simulink model "MyPTControlOSM_RTW"  (Simulink 8.7)
settings: Solver=ode1  SolverMode=SingleTasking  StartTime=0.0  StopTime=inf  FixedStep=0.0002  RelTol=1e-3
PreLoadFcn:
  | vehicle = 'Car'; if ~length(which('cmcmd')), cmenv; end
  | MyPTControlOSM_RTW_bus
InitFcn:
  | vehicle = 'Car'; if ~length(which('cmcmd')), cmenv; end
  | MyPTControlOSM_RTW_bus
undefined symbols (not defined in the file or in its folder): OperationState, OSMFunc, rv, State
libraries: simulink x14
(part 1 of 2)
Description:
  | CarMaker Plug-in Model Target
settings Model: Creator=ml  LastModifiedBy=IPG
settings DataIOCC: SignalLoggingSaveFormat=ModelDataLogs
settings OptimizationCC: ExpressionDepthLimit=2147483647
settings DebuggingCC: FcnCallInpInsideContextMsg=UseLocalSettings  StateNameClashWarn=warning
settings HardwareCC: TargetHWDeviceType=32-bit Generic  ProdEqTarget=off
settings RTWCC: SystemTargetFile=CarMaker.tlc  TemplateMakefile=CarMaker_unix-win64.tmf  Description=CarMaker Plug-in Model Target
settings CodeAppCC: MaxIdLength=63
settings STFCustomTargetCC: ModelReferenceCompliant=off  GeneratePreprocessorConditionals=Disable all  MultiInstanceERTCode=on  CodeInterfacePackaging=Reusable function  CPPClassGenCompliant=on  GRTInterface=off  GenerateAllocFcn=on  SystemTargetFile=CarMaker.tlc
settings GRTTargetCC: ModelReferenceCompliant=off  ParMdlRefBuildCompliant=off  CompOptLevelCompliant=off  ConcurrentExecutionCompliant=off  CombineOutputUpdateFcns=off  MatFileLogging=off  MultiInstanceERTCode=on  CodeInterfacePackaging=Reusable function  GenerateAllocFcn=on  UseToolchainInfoCompliant=off  ExtModeMexFile=noextcomm
settings CustomProperty: DataType=string  Value=..
settings EnumStrPairs: String=Car

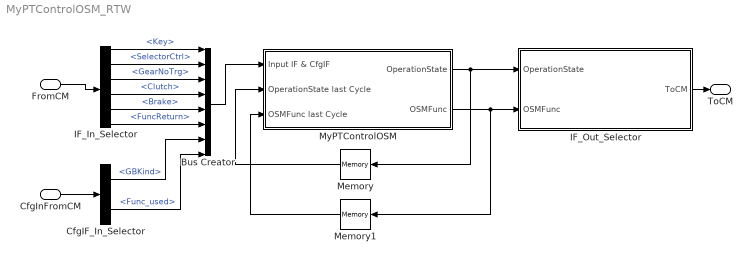
== system MyPTControlOSM_RTW ==
  FromCM : Inport  OutDataTypeStr=Bus: cmPTControlOSMIn
  CfgInFromCM : Inport  Port=2  OutDataTypeStr=Bus: cmPTControlOSMCfgIn
  Bus Creator : BusCreator  Inputs=8
  CfgIF_In_Selector : BusSelector  OutputSignals=GBKind,Func_used
  IF_In_Selector : BusSelector  OutputSignals=Key,SelectorCtrl,GearNoTrg,Clutch,Brake,FuncReturn
  IF_Out_Selector : Subsystem  mask(Signal Selection){}
      mask help: Signal Selection Block
      settings: OpenFcn=cmSignalSelect('SignalSelection_CB',gcb)
  Memory : Memory
  Memory1 : Memory
  MyPTControlOSM : Subsystem
  ToCM : Outport  OutDataTypeStr=Bus: cmPTControlOSMOut
  wires:
  FromCM/1 -> IF_In_Selector/1
  IF_Out_Selector/1(ToCM) -> ToCM/1
  CfgInFromCM/1 -> CfgIF_In_Selector/1
  MyPTControlOSM/1(OperationState) -> Memory/1, IF_Out_Selector/1(OperationState)
  Memory/1 -> MyPTControlOSM/2(OperationState last Cycle)
  IF_In_Selector/1 -> Bus Creator/1  "<Key>"
  IF_In_Selector/2 -> Bus Creator/2  "<SelectorCtrl>"
  IF_In_Selector/3 -> Bus Creator/3  "<GearNoTrg>"
  IF_In_Selector/4 -> Bus Creator/4  "<Clutch>"
  IF_In_Selector/5 -> Bus Creator/5  "<Brake>"
  IF_In_Selector/6 -> Bus Creator/6  "<FuncReturn>"
  CfgIF_In_Selector/1 -> Bus Creator/7  "<GBKind>"
  CfgIF_In_Selector/2 -> Bus Creator/8  "<Func_used>"
  Bus Creator/1 -> MyPTControlOSM/1(Input IF & CfgIF)
  Memory1/1 -> MyPTControlOSM/3(OSMFunc last Cycle)
  MyPTControlOSM/2(OSMFunc) -> Memory1/1, IF_Out_Selector/2(OSMFunc)

== system MyPTControlOSM_RTW/IF_Out_Selector ==
  OperationState : Inport
  OSMFunc : Inport  Port=2
  OperationError : Constant  Value=0
  RateTransition : RateTransition  OutPortSampleTime=str2num(get_param(bdroot,'FixedStep'))
  cmPTControlOSMOut : BusCreator  Inputs=3
  ToCM : Outport
  wires:
  RateTransition/1 -> ToCM/1
  cmPTControlOSMOut/1 -> RateTransition/1
  OperationError/1 -> cmPTControlOSMOut/2  "OperationError"
  OperationState/1 -> cmPTControlOSMOut/1  "OperationState"
  OSMFunc/1 -> cmPTControlOSMOut/3  "OSMFunc"

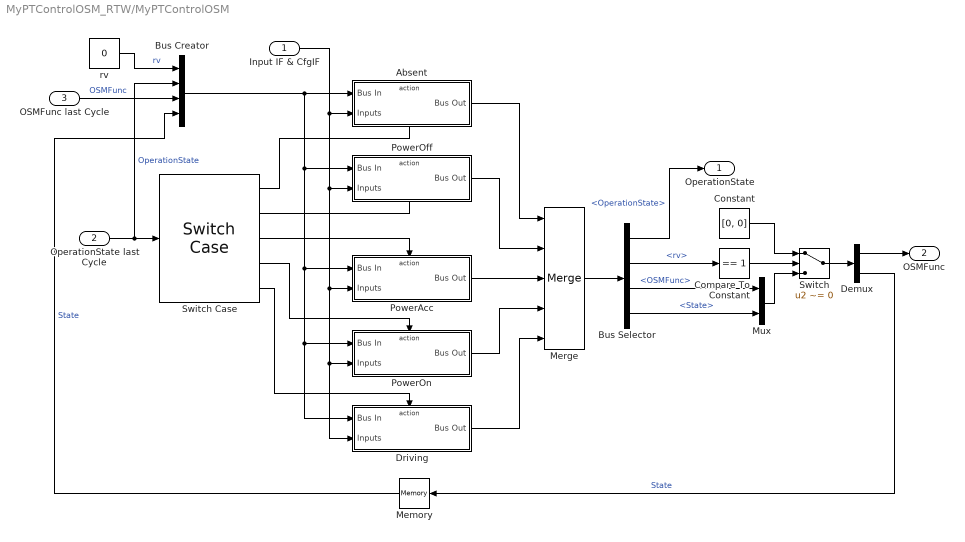
== system MyPTControlOSM_RTW/MyPTControlOSM ==
  Input IF & CfgIF : Inport
  OperationState last Cycle : Inport  Port=2
  OSMFunc last Cycle : Inport  Port=3
  Absent : Subsystem  TreatAsAtomicUnit=on
  Bus Creator : BusCreator  Inputs=4
  Bus Selector : BusSelector  OutputSignals=OperationState,rv,OSMFunc,State
  Compare To Constant : simulink/Logic and Bit Operations/Compare To Constant  SystemSampleTime=-1  relop===  const=1  LogicOutDataTypeMode=uint8  ZeroCross=off
  Constant : Constant  Value=[0, 0]
  Demux : Demux  Outputs=2
  Driving : Subsystem  TreatAsAtomicUnit=on
  Memory : Memory
  Merge : Merge  Inputs=5
  Mux : Mux  Inputs=2
  PowerAcc : Subsystem  TreatAsAtomicUnit=on
  PowerOff : Subsystem  TreatAsAtomicUnit=on
  PowerOn : Subsystem  TreatAsAtomicUnit=on
  Switch : Switch  Criteria=u2 ~= 0
  Switch Case : SwitchCase  CaseConditions={0,1,2,3}
  rv : Constant  Value=0
  OperationState : Outport
  OSMFunc : Outport  Port=2
  wires:
  OperationState last Cycle/1 -> Switch Case/1, Bus Creator/2  "OperationState"
  Switch Case/3 -> PowerAcc/Action
  Switch Case/2 -> PowerOff/Action
  Absent/1(Bus Out) -> Merge/1
  PowerOff/1(Bus Out) -> Merge/2
  PowerAcc/1(Bus Out) -> Merge/3
  rv/1 -> Bus Creator/1  "rv"
  Bus Creator/1 -> Absent/1(Bus In), PowerOff/1(Bus In), PowerAcc/1(Bus In), Driving/1(Bus In), PowerOn/1(Bus In)
  Merge/1 -> Bus Selector/1
  Input IF & CfgIF/1 -> PowerAcc/2(Inputs), Driving/2(Inputs), PowerOn/2(Inputs), PowerOff/2(Inputs), Absent/2(Inputs)
  Bus Selector/1 -> OperationState/1  "<OperationState>"
  Switch/1 -> Demux/1
  Demux/2 -> Memory/1  "State"
  Demux/1 -> OSMFunc/1
  Bus Selector/2 -> Compare To Constant/1  "<rv>"
  Bus Selector/3 -> Mux/1  "<OSMFunc>"
  Bus Selector/4 -> Mux/2  "<State>"
  OSMFunc last Cycle/1 -> Bus Creator/3  "OSMFunc"
  Memory/1 -> Bus Creator/4  "State"
  Driving/1(Bus Out) -> Merge/5
  PowerOn/1(Bus Out) -> Merge/4
  Compare To Constant/1 -> Switch/2
  Constant/1 -> Switch/1
  Mux/1 -> Switch/3
  Switch Case/4 -> PowerOn/Action
  Switch Case/5 -> Driving/Action
  Switch Case/1 -> Absent/Action

== system MyPTControlOSM_RTW/MyPTControlOSM/Absent ==
  Bus In : Inport
  Inputs : Inport  Port=2
  Absent : ActionPort  ActionType=case
  "Absent -> PowerOff?" : Subsystem  TreatAsAtomicUnit=on
  Absent Function exist? : Subsystem  TreatAsAtomicUnit=on
  Bus Selector : BusSelector  OutputSignals=State
  Merge : Merge  Inputs=6
  PowerOff function exist? : Subsystem  TreatAsAtomicUnit=on
  PowerOff reached : Subsystem  TreatAsAtomicUnit=on
  Signal Conversion : SignalConversion  ConversionOutput=Bus copy  OverrideOpt=off
  Switch Case : SwitchCase  CaseConditions={0,1,2,3,4}
  Wait for Absent is ready : Subsystem  TreatAsAtomicUnit=on
  Wait for PowerOff is ready : Subsystem  TreatAsAtomicUnit=on
  Bus Out : Outport
  wires:
  Signal Conversion/1 -> Bus Out/1
  Bus In/1 -> Bus Selector/1, Absent Function exist?/2(Bus In), Wait for Absent is ready/1(Bus In), "Absent -> PowerOff?"/1(Bus In), PowerOff reached/1(Bus In), Wait for PowerOff is ready/1(Bus In), PowerOff function exist?/1(Bus In)
  Bus Selector/1 -> Switch Case/1  "<State>"
  Switch Case/2 -> Wait for Absent is ready/Action
  Switch Case/5 -> Wait for PowerOff is ready/Action
  Switch Case/6 -> PowerOff reached/Action
  Switch Case/3 -> "Absent -> PowerOff?"/Action
  Switch Case/4 -> PowerOff function exist?/Action
  Absent Function exist?/1(Bus Out) -> Merge/1
  Wait for Absent is ready/1(Bus Out) -> Merge/2
  "Absent -> PowerOff?"/1(Bus Out) -> Merge/3
  Wait for PowerOff is ready/1(Bus Out) -> Merge/5
  PowerOff reached/1(Bus Out) -> Merge/6
  Merge/1 -> Signal Conversion/1
  Inputs/1 -> Absent Function exist?/1(Input), Wait for Absent is ready/2(Input), "Absent -> PowerOff?"/2(Input), PowerOff function exist?/2(Input), Wait for PowerOff is ready/2(Input)
  PowerOff function exist?/1(Bus Out) -> Merge/4
  Switch Case/1 -> Absent Function exist?/Action

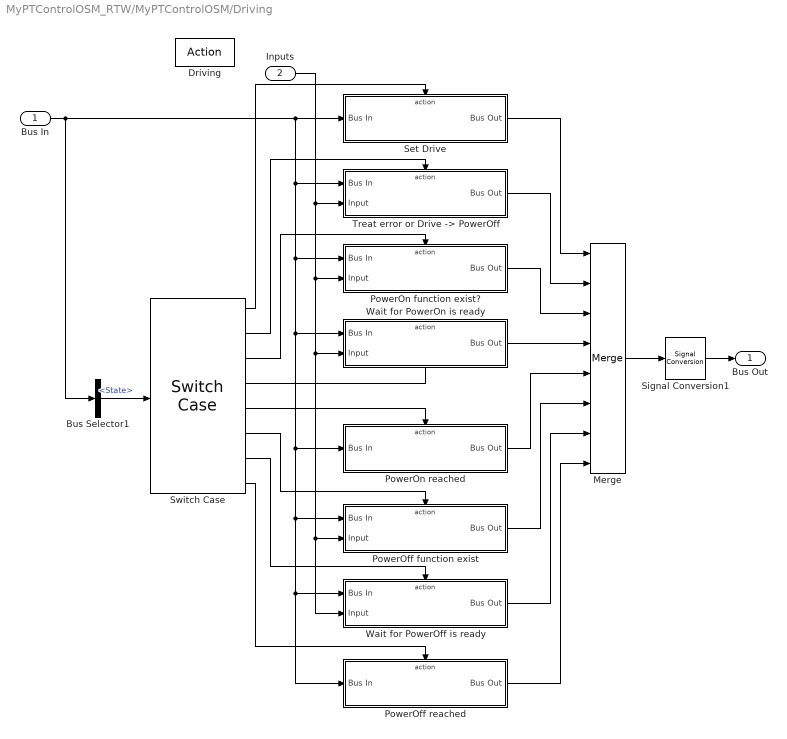
== system MyPTControlOSM_RTW/MyPTControlOSM/Driving ==
  Bus In : Inport
  Inputs : Inport  Port=2
  Driving : ActionPort  ActionType=default
  Bus Selector1 : BusSelector  OutputSignals=State
  Merge : Merge  Inputs=8
  PowerOff function exist : Subsystem  TreatAsAtomicUnit=on
  PowerOff reached : Subsystem  TreatAsAtomicUnit=on
  PowerOn function exist? : Subsystem  TreatAsAtomicUnit=on
  PowerOn reached : Subsystem  TreatAsAtomicUnit=on
  Set Drive : Subsystem  TreatAsAtomicUnit=on
  Signal Conversion1 : SignalConversion  ConversionOutput=Bus copy  OverrideOpt=off
  Switch Case : SwitchCase  CaseConditions={0,1,2,3,4,5,6}
  "Treat error or Drive -> PowerOff" : Subsystem  TreatAsAtomicUnit=on
  Wait for PowerOff is ready : Subsystem  TreatAsAtomicUnit=on
  Wait for PowerOn is ready : Subsystem  TreatAsAtomicUnit=on
  Bus Out : Outport
  wires:
  Signal Conversion1/1 -> Bus Out/1
  Bus Selector1/1 -> Switch Case/1  "<State>"
  Switch Case/3 -> PowerOn function exist?/Action
  Merge/1 -> Signal Conversion1/1
  Switch Case/8 -> PowerOff reached/Action
  Switch Case/1 -> Set Drive/Action
  Switch Case/2 -> "Treat error or Drive -> PowerOff"/Action
  Bus In/1 -> Bus Selector1/1, "Treat error or Drive -> PowerOff"/1(Bus In), Wait for PowerOn is ready/1(Bus In), PowerOn reached/1(Bus In), PowerOff reached/1(Bus In), Wait for PowerOff is ready/1(Bus In), PowerOff function exist/1(Bus In), PowerOn function exist?/1(Bus In), Set Drive/1(Bus In)
  Inputs/1 -> Wait for PowerOn is ready/2(Input), Wait for PowerOff is ready/2(Input), PowerOff function exist/2(Input), PowerOn function exist?/2(Input), "Treat error or Drive -> PowerOff"/2(Input)
  Switch Case/4 -> Wait for PowerOn is ready/Action
  Switch Case/5 -> PowerOn reached/Action
  Switch Case/6 -> PowerOff function exist/Action
  Switch Case/7 -> Wait for PowerOff is ready/Action
  Set Drive/1(Bus Out) -> Merge/1
  "Treat error or Drive -> PowerOff"/1(Bus Out) -> Merge/2
  Wait for PowerOn is ready/1(Bus Out) -> Merge/4
  Wait for PowerOff is ready/1(Bus Out) -> Merge/7
  PowerOff reached/1(Bus Out) -> Merge/8
  PowerOn reached/1(Bus Out) -> Merge/5
  PowerOn function exist?/1(Bus Out) -> Merge/3
  PowerOff function exist/1(Bus Out) -> Merge/6

== system MyPTControlOSM_RTW/MyPTControlOSM/PowerAcc ==
  Bus In : Inport
  Inputs : Inport  Port=2
  PowerAcc : ActionPort  ActionType=case
  Bus Selector1 : BusSelector  OutputSignals=State
  Merge : Merge  Inputs=4
  "PowerAcc -> PowerOn?" : Subsystem  TreatAsAtomicUnit=on
  PowerOn function exist? : Subsystem  TreatAsAtomicUnit=on
  PowerOn reached : Subsystem  TreatAsAtomicUnit=on
  Signal Conversion : SignalConversion  ConversionOutput=Bus copy  OverrideOpt=off
  Switch Case : SwitchCase  CaseConditions={0,1,2}
  Wait for PowerOn is ready : Subsystem  TreatAsAtomicUnit=on
  Bus Out : Outport
  wires:
  Signal Conversion/1 -> Bus Out/1
  Bus Selector1/1 -> Switch Case/1  "<State>"
  Switch Case/3 -> Wait for PowerOn is ready/Action
  Wait for PowerOn is ready/1(Bus Out) -> Merge/3
  Merge/1 -> Signal Conversion/1
  Switch Case/4 -> PowerOn reached/Action
  Switch Case/1 -> "PowerAcc -> PowerOn?"/Action
  Switch Case/2 -> PowerOn function exist?/Action
  "PowerAcc -> PowerOn?"/1(Bus Out) -> Merge/1
  PowerOn reached/1(Bus Out) -> Merge/4
  PowerOn function exist?/1(Bus Out) -> Merge/2
  Bus In/1 -> Bus Selector1/1, "PowerAcc -> PowerOn?"/1(Bus In), PowerOn reached/1(Bus In), Wait for PowerOn is ready/1(Bus In), PowerOn function exist?/1(Bus In)
  Inputs/1 -> Wait for PowerOn is ready/2(Input), PowerOn function exist?/2(Input), "PowerAcc -> PowerOn?"/2(Input)

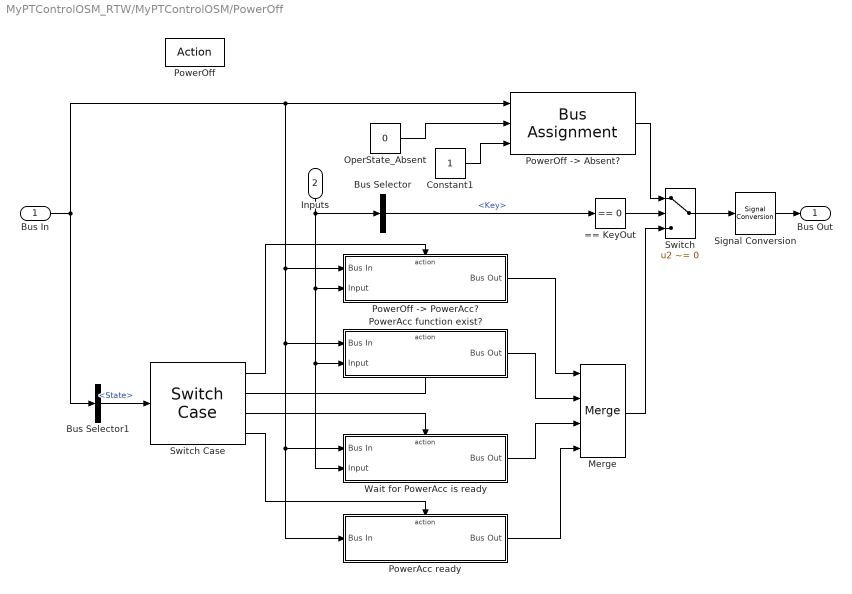
== system MyPTControlOSM_RTW/MyPTControlOSM/PowerOff ==
  Bus In : Inport
  Inputs : Inport  Port=2
  PowerOff : ActionPort  ActionType=case
  == KeyOut : simulink/Logic and Bit Operations/Compare To Zero  SystemSampleTime=-1  relop===  LogicOutDataTypeMode=uint8  ZeroCross=off
  Bus Selector : BusSelector  OutputSignals=Key
  Bus Selector1 : BusSelector  OutputSignals=State
  Constant1 : Constant
  Merge : Merge  Inputs=4
  OperState_Absent : Constant  Value=0
  PowerAcc function exist? : Subsystem  TreatAsAtomicUnit=on
  PowerAcc ready : Subsystem  TreatAsAtomicUnit=on
  "PowerOff -> Absent?" : BusAssignment  AssignedSignals=OperationState,rv
  "PowerOff -> PowerAcc?" : Subsystem  TreatAsAtomicUnit=on
  Signal Conversion : SignalConversion  ConversionOutput=Bus copy  OverrideOpt=off
  Switch : Switch  Criteria=u2 ~= 0
  Switch Case : SwitchCase  CaseConditions={0,1,2}
  Wait for PowerAcc is ready : Subsystem  TreatAsAtomicUnit=on
  Bus Out : Outport
  wires:
  Signal Conversion/1 -> Bus Out/1
  Switch/1 -> Signal Conversion/1
  Inputs/1 -> Bus Selector/1, "PowerOff -> PowerAcc?"/2(Input), Wait for PowerAcc is ready/2(Input), PowerAcc function exist?/2(Input)
  Bus Selector/1 -> == KeyOut/1  "<Key>"
  == KeyOut/1 -> Switch/2
  "PowerOff -> Absent?"/1 -> Switch/1
  Bus In/1 -> Bus Selector1/1, "PowerOff -> Absent?"/1, "PowerOff -> PowerAcc?"/1(Bus In), Wait for PowerAcc is ready/1(Bus In), PowerAcc ready/1(Bus In), PowerAcc function exist?/1(Bus In)
  OperState_Absent/1 -> "PowerOff -> Absent?"/2
  Constant1/1 -> "PowerOff -> Absent?"/3
  Bus Selector1/1 -> Switch Case/1  "<State>"
  Switch Case/3 -> Wait for PowerAcc is ready/Action
  Wait for PowerAcc is ready/1(Bus Out) -> Merge/3
  Merge/1 -> Switch/3
  Switch Case/4 -> PowerAcc ready/Action
  Switch Case/1 -> "PowerOff -> PowerAcc?"/Action
  Switch Case/2 -> PowerAcc function exist?/Action
  "PowerOff -> PowerAcc?"/1(Bus Out) -> Merge/1
  PowerAcc ready/1(Bus Out) -> Merge/4
  PowerAcc function exist?/1(Bus Out) -> Merge/2

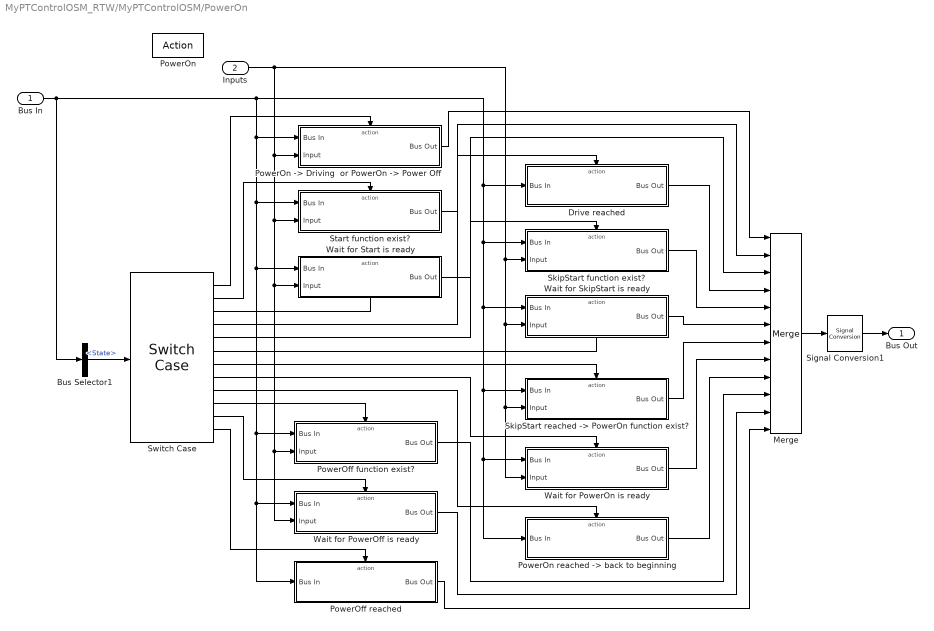
== system MyPTControlOSM_RTW/MyPTControlOSM/PowerOn ==
  Bus In : Inport
  Inputs : Inport  Port=2
  PowerOn : ActionPort  ActionType=case
  Bus Selector1 : BusSelector  OutputSignals=State
  Drive reached : Subsystem  TreatAsAtomicUnit=on
  Merge : Merge  Inputs=12
  PowerOff function exist? : Subsystem  TreatAsAtomicUnit=on
  PowerOff reached : Subsystem  TreatAsAtomicUnit=on
  "PowerOn -> Driving  or PowerOn -> Power Off" : Subsystem  TreatAsAtomicUnit=on
  "PowerOn reached -> back to beginning" : Subsystem  TreatAsAtomicUnit=on
  Signal Conversion1 : SignalConversion  ConversionOutput=Bus copy  OverrideOpt=off
  SkipStart function exist? : Subsystem  TreatAsAtomicUnit=on
  "SkipStart reached -> PowerOn function exist?" : Subsystem  TreatAsAtomicUnit=on
  Start function exist? : Subsystem  TreatAsAtomicUnit=on
  Switch Case : SwitchCase  CaseConditions={0,1,2,3,4,5,6,7,8,9,10}
  Wait for PowerOff is ready : Subsystem  TreatAsAtomicUnit=on
  Wait for PowerOn is ready : Subsystem  TreatAsAtomicUnit=on
  Wait for SkipStart is ready : Subsystem  TreatAsAtomicUnit=on
  Wait for Start is ready : Subsystem  TreatAsAtomicUnit=on
  Bus Out : Outport
  wires:
  Signal Conversion1/1 -> Bus Out/1
  Bus Selector1/1 -> Switch Case/1  "<State>"
  Merge/1 -> Signal Conversion1/1
  Bus In/1 -> Bus Selector1/1, "PowerOn reached -> back to beginning"/1(Bus In), Wait for PowerOn is ready/1(Bus In), "SkipStart reached -> PowerOn function exist?"/1(Bus In), Wait for SkipStart is ready/1(Bus In), SkipStart function exist?/1(Bus In), Drive reached/1(Bus In), Start function exist?/1(Bus In), PowerOff reached/1(Bus In), Wait for PowerOff is ready/1(Bus In), PowerOff function exist?/1(Bus In), Wait for Start is ready/1(Bus In), "PowerOn -> Driving  or PowerOn -> Power Off"/1(Bus In)
  Switch Case/1 -> "PowerOn -> Driving  or PowerOn -> Power Off"/Action
  Switch Case/2 -> Start function exist?/Action
  Switch Case/3 -> Wait for Start is ready/Action
  Switch Case/4 -> Drive reached/Action
  Switch Case/5 -> SkipStart function exist?/Action
  Switch Case/6 -> Wait for SkipStart is ready/Action
  Switch Case/7 -> "SkipStart reached -> PowerOn function exist?"/Action
  Switch Case/8 -> Wait for PowerOn is ready/Action
  Switch Case/9 -> "PowerOn reached -> back to beginning"/Action
  Switch Case/10 -> PowerOff function exist?/Action
  Switch Case/11 -> Wait for PowerOff is ready/Action
  Switch Case/12 -> PowerOff reached/Action
  "PowerOn -> Driving  or PowerOn -> Power Off"/1(Bus Out) -> Merge/1
  Start function exist?/1(Bus Out) -> Merge/2
  Wait for Start is ready/1(Bus Out) -> Merge/3
  Drive reached/1(Bus Out) -> Merge/4
  SkipStart function exist?/1(Bus Out) -> Merge/5
  Wait for SkipStart is ready/1(Bus Out) -> Merge/6
  "SkipStart reached -> PowerOn function exist?"/1(Bus Out) -> Merge/7
  Wait for PowerOn is ready/1(Bus Out) -> Merge/8
  "PowerOn reached -> back to beginning"/1(Bus Out) -> Merge/9
  PowerOff function exist?/1(Bus Out) -> Merge/10
  Wait for PowerOff is ready/1(Bus Out) -> Merge/11
  PowerOff reached/1(Bus Out) -> Merge/12
  Inputs/1 -> SkipStart function exist?/2(Input), Wait for PowerOn is ready/2(Input), "SkipStart reached -> PowerOn function exist?"/2(Input), Wait for SkipStart is ready/2(Input), Start function exist?/2(Input), Wait for PowerOff is ready/2(Input), PowerOff function exist?/2(Input), Wait for Start is ready/2(Input), "PowerOn -> Driving  or PowerOn -> Power Off"/2(Input)

== system MyPTControlOSM_RTW/MyPTControlOSM/Absent/Absent -> PowerOff? ==
  Bus In : Inport
  Input : Inport  Port=2
  "State 2 Absent -> PowerOff?" : ActionPort  ActionType=case
  >= KeyIn_PowerOff : simulink/Logic and Bit Operations/Compare To Constant  SystemSampleTime=-1  relop=>=  const=1  LogicOutDataTypeMode=uint8  ZeroCross=off
  Bus Assignment : BusAssignment  AssignedSignals=OSMFunc,State
  Bus Selector : BusSelector  OutputSignals=Key
  Constant : Constant  Value=3
  Constant1 : Constant  Value=2
  OSMFunc_None : Constant  Value=0
  Signal Conversion : SignalConversion  ConversionOutput=Bus copy  OverrideOpt=off
  Switch : Switch  Criteria=u2 ~= 0
  Bus Out : Outport
  wires:
  Signal Conversion/1 -> Bus Out/1
  Bus Assignment/1 -> Signal Conversion/1
  Bus In/1 -> Bus Assignment/1
  OSMFunc_None/1 -> Bus Assignment/2
  Switch/1 -> Bus Assignment/3
  Input/1 -> Bus Selector/1
  Bus Selector/1 -> >= KeyIn_PowerOff/1  "<Key>"
  >= KeyIn_PowerOff/1 -> Switch/2
  Constant/1 -> Switch/1
  Constant1/1 -> Switch/3

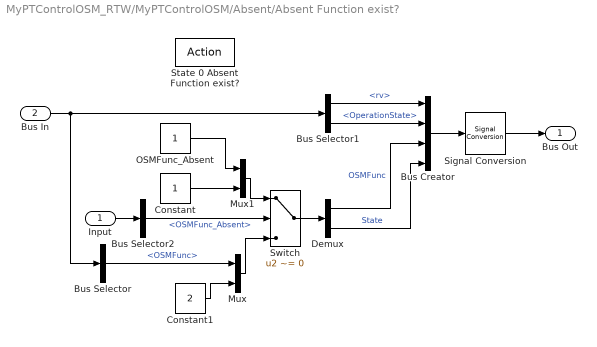
== system MyPTControlOSM_RTW/MyPTControlOSM/Absent/Absent Function exist? ==
  Input : Inport
  Bus In : Inport  Port=2
  State 0 Absent Function exist? : ActionPort  ActionType=case
  Bus Creator : BusCreator  Inputs=4
  Bus Selector : BusSelector  OutputSignals=OSMFunc
  Bus Selector1 : BusSelector  OutputSignals=rv,OperationState
  Bus Selector2 : BusSelector  OutputSignals=Func_used.OSMFunc_Absent
  Constant : Constant
  Constant1 : Constant  Value=2
  Demux : Demux  Outputs=2
  Mux : Mux  Inputs=2
  Mux1 : Mux  Inputs=2
  OSMFunc_Absent : Constant
  Signal Conversion : SignalConversion  ConversionOutput=Bus copy  OverrideOpt=off
  Switch : Switch  Criteria=u2 ~= 0
  Bus Out : Outport
  wires:
  Bus In/1 -> Bus Selector/1, Bus Selector1/1
  Bus Creator/1 -> Signal Conversion/1
  Input/1 -> Bus Selector2/1
  Switch/1 -> Demux/1
  Mux/1 -> Switch/3
  Bus Selector/1 -> Mux/1  "<OSMFunc>"
  Constant1/1 -> Mux/2
  Bus Selector1/1 -> Bus Creator/1  "<rv>"
  Signal Conversion/1 -> Bus Out/1
  Bus Selector1/2 -> Bus Creator/2  "<OperationState>"
  Demux/1 -> Bus Creator/3  "OSMFunc"
  Demux/2 -> Bus Creator/4  "State"
  Bus Selector2/1 -> Switch/2  "<OSMFunc_Absent>"
  Mux1/1 -> Switch/1
  OSMFunc_Absent/1 -> Mux1/1
  Constant/1 -> Mux1/2

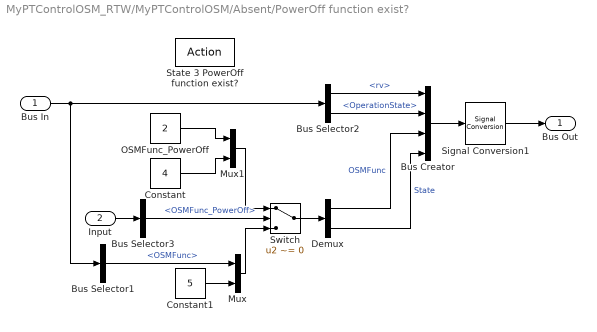
== system MyPTControlOSM_RTW/MyPTControlOSM/Absent/PowerOff function exist? ==
  Bus In : Inport
  Input : Inport  Port=2
  State 3 PowerOff function exist? : ActionPort  ActionType=case
  Bus Creator : BusCreator  Inputs=4
  Bus Selector1 : BusSelector  OutputSignals=OSMFunc
  Bus Selector2 : BusSelector  OutputSignals=rv,OperationState
  Bus Selector3 : BusSelector  OutputSignals=Func_used.OSMFunc_PowerOff
  Constant : Constant  Value=4
  Constant1 : Constant  Value=5
  Demux : Demux  Outputs=2
  Mux : Mux  Inputs=2
  Mux1 : Mux  Inputs=2
  OSMFunc_PowerOff : Constant  Value=2
  Signal Conversion1 : SignalConversion  ConversionOutput=Bus copy  OverrideOpt=off
  Switch : Switch  Criteria=u2 ~= 0
  Bus Out : Outport
  wires:
  Bus In/1 -> Bus Selector1/1, Bus Selector2/1
  Bus Creator/1 -> Signal Conversion1/1
  Input/1 -> Bus Selector3/1
  Switch/1 -> Demux/1
  Mux/1 -> Switch/3
  Bus Selector1/1 -> Mux/1  "<OSMFunc>"
  Constant1/1 -> Mux/2
  Bus Selector2/1 -> Bus Creator/1  "<rv>"
  Signal Conversion1/1 -> Bus Out/1
  Bus Selector2/2 -> Bus Creator/2  "<OperationState>"
  Demux/1 -> Bus Creator/3  "OSMFunc"
  Demux/2 -> Bus Creator/4  "State"
  Bus Selector3/1 -> Switch/2  "<OSMFunc_PowerOff>"
  Mux1/1 -> Switch/1
  OSMFunc_PowerOff/1 -> Mux1/1
  Constant/1 -> Mux1/2

== system MyPTControlOSM_RTW/MyPTControlOSM/Absent/PowerOff reached ==
  Bus In : Inport
  State 5 PowerOff reached : ActionPort  ActionType=default
  Bus Creator : BusCreator  Inputs=4
  Bus Selector2 : BusSelector  OutputSignals=OSMFunc,State
  Constant : Constant
  OperState_PowerOff : Constant
  Signal Conversion : SignalConversion  ConversionOutput=Bus copy  OverrideOpt=off
  Bus Out : Outport
  wires:
  Signal Conversion/1 -> Bus Out/1
  Bus Selector2/2 -> Bus Creator/4  "<State>"
  Bus Selector2/1 -> Bus Creator/3  "<OSMFunc>"
  OperState_PowerOff/1 -> Bus Creator/2  "OperationState"
  Constant/1 -> Bus Creator/1  "rv"
  Bus Creator/1 -> Signal Conversion/1
  Bus In/1 -> Bus Selector2/1

== system MyPTControlOSM_RTW/MyPTControlOSM/Absent/Wait for Absent is ready ==
  Bus In : Inport
  Input : Inport  Port=2
  State 1 Wait for Absent is ready : ActionPort  ActionType=case
  Bus Assignment : BusAssignment  AssignedSignals=State
  Bus Selector : BusSelector  OutputSignals=FuncReturn
  Constant : Constant  Value=2
  Constant1 : Constant
  Signal Conversion : SignalConversion  ConversionOutput=Bus copy  OverrideOpt=off
  Switch : Switch  Criteria=u2 ~= 0
  Bus Out : Outport
  wires:
  Bus In/1 -> Bus Assignment/1
  Bus Assignment/1 -> Signal Conversion/1
  Signal Conversion/1 -> Bus Out/1
  Switch/1 -> Bus Assignment/2
  Input/1 -> Bus Selector/1
  Bus Selector/1 -> Switch/2  "<FuncReturn>"
  Constant/1 -> Switch/1
  Constant1/1 -> Switch/3

== system MyPTControlOSM_RTW/MyPTControlOSM/Absent/Wait for PowerOff is ready ==
  Bus In : Inport
  Input : Inport  Port=2
  State 4 Wait for PowerOff is ready : ActionPort  ActionType=case
  Bus Assignment : BusAssignment  AssignedSignals=State
  Bus Selector : BusSelector  OutputSignals=FuncReturn
  Constant : Constant  Value=5
  Constant1 : Constant  Value=4
  Signal Conversion : SignalConversion  ConversionOutput=Bus copy  OverrideOpt=off
  Switch : Switch  Criteria=u2 ~= 0
  Bus Out : Outport
  wires:
  Signal Conversion/1 -> Bus Out/1
  Input/1 -> Bus Selector/1
  Bus Assignment/1 -> Signal Conversion/1
  Bus In/1 -> Bus Assignment/1
  Bus Selector/1 -> Switch/2  "<FuncReturn>"
  Switch/1 -> Bus Assignment/2
  Constant/1 -> Switch/1
  Constant1/1 -> Switch/3

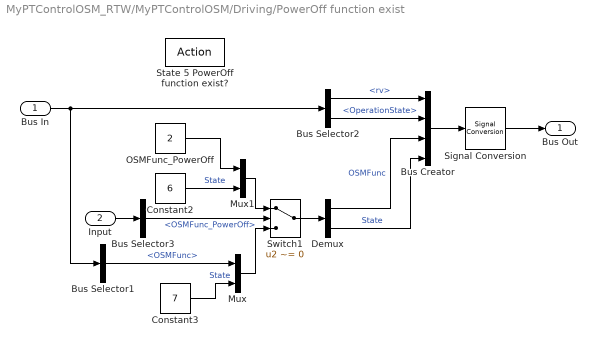
== system MyPTControlOSM_RTW/MyPTControlOSM/Driving/PowerOff function exist ==
  Bus In : Inport
  Input : Inport  Port=2
  State 5 PowerOff function exist? : ActionPort  ActionType=case
  Bus Creator : BusCreator  Inputs=4
  Bus Selector1 : BusSelector  OutputSignals=OSMFunc
  Bus Selector2 : BusSelector  OutputSignals=rv,OperationState
  Bus Selector3 : BusSelector  OutputSignals=Func_used.OSMFunc_PowerOff
  Constant2 : Constant  Value=6
  Constant3 : Constant  Value=7
  Demux : Demux  Outputs=2
  Mux : Mux  Inputs=2
  Mux1 : Mux  Inputs=2
  OSMFunc_PowerOff : Constant  Value=2
  Signal Conversion : SignalConversion  ConversionOutput=Bus copy  OverrideOpt=off
  Switch1 : Switch  Criteria=u2 ~= 0
  Bus Out : Outport
  wires:
  Bus In/1 -> Bus Selector1/1, Bus Selector2/1
  Bus Creator/1 -> Signal Conversion/1
  Input/1 -> Bus Selector3/1
  Switch1/1 -> Demux/1
  Mux/1 -> Switch1/3
  Bus Selector1/1 -> Mux/1  "<OSMFunc>"
  Constant3/1 -> Mux/2  "State"
  Signal Conversion/1 -> Bus Out/1
  Bus Selector2/2 -> Bus Creator/2  "<OperationState>"
  Demux/1 -> Bus Creator/3  "OSMFunc"
  Demux/2 -> Bus Creator/4  "State"
  Bus Selector3/1 -> Switch1/2  "<OSMFunc_PowerOff>"
  Constant2/1 -> Mux1/2  "State"
  OSMFunc_PowerOff/1 -> Mux1/1
  Mux1/1 -> Switch1/1
  Bus Selector2/1 -> Bus Creator/1  "<rv>"

== system MyPTControlOSM_RTW/MyPTControlOSM/Driving/PowerOff reached ==
  Bus In : Inport
  State 7 PowerOff reached : ActionPort  ActionType=default
  Bus Creator : BusCreator  Inputs=4
  Bus Selector2 : BusSelector  OutputSignals=OSMFunc,State
  Constant : Constant
  OperState_PowerOff : Constant
  Signal Conversion : SignalConversion  ConversionOutput=Bus copy  OverrideOpt=off
  Bus Out : Outport
  wires:
  Signal Conversion/1 -> Bus Out/1
  Bus Selector2/2 -> Bus Creator/4  "<State>"
  Bus Selector2/1 -> Bus Creator/3  "<OSMFunc>"
  OperState_PowerOff/1 -> Bus Creator/2  "OperationState"
  Constant/1 -> Bus Creator/1  "rv"
  Bus Creator/1 -> Signal Conversion/1
  Bus In/1 -> Bus Selector2/1

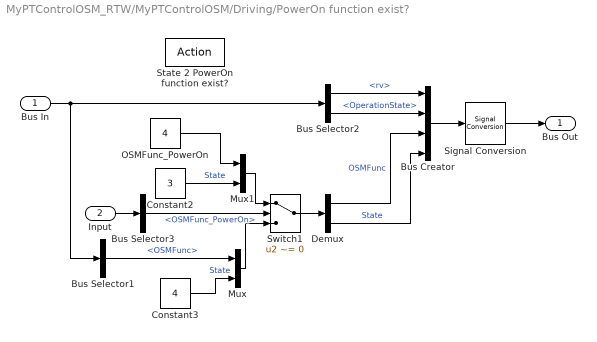
== system MyPTControlOSM_RTW/MyPTControlOSM/Driving/PowerOn function exist? ==
  Bus In : Inport
  Input : Inport  Port=2
  State 2 PowerOn function exist? : ActionPort  ActionType=case
  Bus Creator : BusCreator  Inputs=4
  Bus Selector1 : BusSelector  OutputSignals=OSMFunc
  Bus Selector2 : BusSelector  OutputSignals=rv,OperationState
  Bus Selector3 : BusSelector  OutputSignals=Func_used.OSMFunc_PowerOn
  Constant2 : Constant  Value=3
  Constant3 : Constant  Value=4
  Demux : Demux  Outputs=2
  Mux : Mux  Inputs=2
  Mux1 : Mux  Inputs=2
  OSMFunc_PowerOn : Constant  Value=4
  Signal Conversion : SignalConversion  ConversionOutput=Bus copy  OverrideOpt=off
  Switch1 : Switch  Criteria=u2 ~= 0
  Bus Out : Outport
  wires:
  Bus In/1 -> Bus Selector1/1, Bus Selector2/1
  Bus Creator/1 -> Signal Conversion/1
  Input/1 -> Bus Selector3/1
  Switch1/1 -> Demux/1
  Mux/1 -> Switch1/3
  Bus Selector1/1 -> Mux/1  "<OSMFunc>"
  Constant3/1 -> Mux/2  "State"
  Signal Conversion/1 -> Bus Out/1
  Bus Selector2/2 -> Bus Creator/2  "<OperationState>"
  Demux/1 -> Bus Creator/3  "OSMFunc"
  Demux/2 -> Bus Creator/4  "State"
  Bus Selector3/1 -> Switch1/2  "<OSMFunc_PowerOn>"
  Bus Selector2/1 -> Bus Creator/1  "<rv>"
  Constant2/1 -> Mux1/2  "State"
  OSMFunc_PowerOn/1 -> Mux1/1
  Mux1/1 -> Switch1/1

== system MyPTControlOSM_RTW/MyPTControlOSM/Driving/PowerOn reached ==
  Bus In : Inport
  State 4 PowerOn reached : ActionPort  ActionType=case
  Bus Creator : BusCreator  Inputs=4
  Bus Selector2 : BusSelector  OutputSignals=OSMFunc,State
  Constant : Constant
  OperState_PowerOn : Constant  Value=3
  Signal Conversion : SignalConversion  ConversionOutput=Bus copy  OverrideOpt=off
  Bus Out : Outport
  wires:
  Signal Conversion/1 -> Bus Out/1
  Bus Selector2/2 -> Bus Creator/4  "<State>"
  Bus Selector2/1 -> Bus Creator/3  "<OSMFunc>"
  OperState_PowerOn/1 -> Bus Creator/2  "OperationState"
  Constant/1 -> Bus Creator/1  "rv"
  Bus Creator/1 -> Signal Conversion/1
  Bus In/1 -> Bus Selector2/1

== system MyPTControlOSM_RTW/MyPTControlOSM/Driving/Set Drive ==
  Bus In : Inport
  State 0 Set Drive : ActionPort  ActionType=case
  Bus Creator : BusCreator  Inputs=4
  Bus Selector1 : BusSelector  OutputSignals=rv,OperationState
  Constant1 : Constant
  OSMFunc_Drive : Constant  Value=7
  Signal Conversion : SignalConversion  ConversionOutput=Bus copy  OverrideOpt=off
  Bus Out : Outport
  wires:
  Bus In/1 -> Bus Selector1/1
  Bus Creator/1 -> Signal Conversion/1
  Bus Selector1/1 -> Bus Creator/1  "<rv>"
  Signal Conversion/1 -> Bus Out/1
  Bus Selector1/2 -> Bus Creator/2  "<OperationState>"
  OSMFunc_Drive/1 -> Bus Creator/3  "OSMFunc"
  Constant1/1 -> Bus Creator/4  "State"

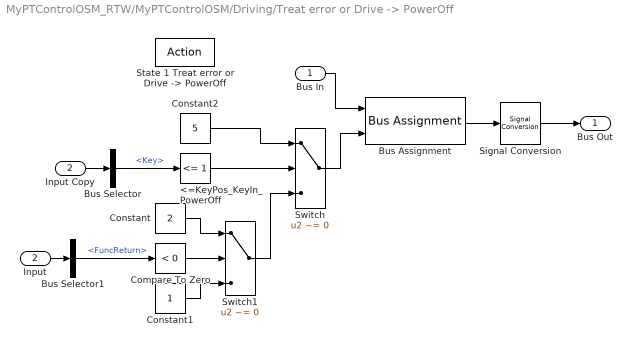
== system MyPTControlOSM_RTW/MyPTControlOSM/Driving/Treat error or Drive -> PowerOff ==
  Bus In : Inport
  Input : Inport  Port=2
  "State 1 Treat error or Drive -> PowerOff" : ActionPort  ActionType=case
  <=KeyPos_KeyIn_PowerOff : simulink/Logic and Bit Operations/Compare To Constant  SystemSampleTime=-1  relop=<=  const=1  LogicOutDataTypeMode=uint8  ZeroCross=off
  Bus Assignment : BusAssignment  AssignedSignals=State
  Bus Selector : BusSelector  OutputSignals=Key
  Bus Selector1 : BusSelector  OutputSignals=FuncReturn
  Compare To Zero : simulink/Logic and Bit Operations/Compare To Zero  SystemSampleTime=-1  relop=<  LogicOutDataTypeMode=uint8  ZeroCross=off
  Constant : Constant  Value=2
  Constant1 : Constant
  Constant2 : Constant  Value=5
  Input Copy : InportShadow  Port=2
  Signal Conversion : SignalConversion  ConversionOutput=Bus copy  OverrideOpt=off
  Switch : Switch  Criteria=u2 ~= 0
  Switch1 : Switch  Criteria=u2 ~= 0
  Bus Out : Outport
  wires:
  Bus Assignment/1 -> Signal Conversion/1
  Signal Conversion/1 -> Bus Out/1
  Bus In/1 -> Bus Assignment/1
  Switch1/1 -> Switch/3
  Switch/1 -> Bus Assignment/2
  Compare To Zero/1 -> Switch1/2
  Constant/1 -> Switch1/1
  Constant1/1 -> Switch1/3
  <=KeyPos_KeyIn_PowerOff/1 -> Switch/2
  Input Copy/1 -> Bus Selector/1
  Input/1 -> Bus Selector1/1
  Bus Selector1/1 -> Compare To Zero/1  "<FuncReturn>"
  Bus Selector/1 -> <=KeyPos_KeyIn_PowerOff/1  "<Key>"
  Constant2/1 -> Switch/1

== system MyPTControlOSM_RTW/MyPTControlOSM/Driving/Wait for PowerOff is ready ==
  Bus In : Inport
  Input : Inport  Port=2
  State 6 Wait for PowerOff is ready : ActionPort  ActionType=case
  Bus Assignment : BusAssignment  AssignedSignals=State
  Bus Selector : BusSelector  OutputSignals=FuncReturn
  Constant : Constant  Value=7
  Constant1 : Constant  Value=6
  Signal Conversion : SignalConversion  ConversionOutput=Bus copy  OverrideOpt=off
  Switch : Switch  Criteria=u2 ~= 0
  Bus Out : Outport
  wires:
  Constant1/1 -> Switch/3
  Constant/1 -> Switch/1
  Bus Selector/1 -> Switch/2  "<FuncReturn>"
  Input/1 -> Bus Selector/1
  Bus In/1 -> Bus Assignment/1
  Bus Assignment/1 -> Signal Conversion/1
  Signal Conversion/1 -> Bus Out/1
  Switch/1 -> Bus Assignment/2

== system MyPTControlOSM_RTW/MyPTControlOSM/Driving/Wait for PowerOn is ready ==
  Bus In : Inport
  Input : Inport  Port=2
  State 3 Wait for PowerOn is ready : ActionPort  ActionType=case
  Bus Assignment : BusAssignment  AssignedSignals=State
  Bus Selector : BusSelector  OutputSignals=FuncReturn
  Constant : Constant  Value=4
  Constant1 : Constant  Value=3
  Signal Conversion : SignalConversion  ConversionOutput=Bus copy  OverrideOpt=off
  Switch : Switch  Criteria=u2 ~= 0
  Bus Out : Outport
  wires:
  Signal Conversion/1 -> Bus Out/1
  Bus Assignment/1 -> Signal Conversion/1
  Bus In/1 -> Bus Assignment/1
  Input/1 -> Bus Selector/1
  Bus Selector/1 -> Switch/2  "<FuncReturn>"
  Constant/1 -> Switch/1
  Constant1/1 -> Switch/3
  Switch/1 -> Bus Assignment/2

== system MyPTControlOSM_RTW/MyPTControlOSM/PowerAcc/PowerAcc -> PowerOn? ==
  Bus In : Inport
  Input : Inport  Port=2
  "State 0 PowerAcc -> PowerOn?" : ActionPort  ActionType=case
  Bus Assignment : BusAssignment  AssignedSignals=State
  Bus Selector : BusSelector  OutputSignals=Key
  Compare To Constant : simulink/Logic and Bit Operations/Compare To Constant  SystemSampleTime=-1  relop=>=  const=3  LogicOutDataTypeMode=uint8  ZeroCross=off
  Constant : Constant
  Constant1 : Constant  Value=0
  Signal Conversion : SignalConversion  ConversionOutput=Bus copy  OverrideOpt=off
  Switch : Switch  Criteria=u2 ~= 0
  Bus Out : Outport
  wires:
  Bus In/1 -> Bus Assignment/1
  Bus Assignment/1 -> Signal Conversion/1
  Signal Conversion/1 -> Bus Out/1
  Switch/1 -> Bus Assignment/2
  Input/1 -> Bus Selector/1
  Bus Selector/1 -> Compare To Constant/1  "<Key>"
  Constant/1 -> Switch/1
  Constant1/1 -> Switch/3
  Compare To Constant/1 -> Switch/2

== system MyPTControlOSM_RTW/MyPTControlOSM/PowerAcc/PowerOn function exist? ==
  Bus In : Inport
  Input : Inport  Port=2
  State 1 PowerOn function exist? : ActionPort  ActionType=case
  Bus Creator : BusCreator  Inputs=4
  Bus Selector : BusSelector  OutputSignals=OSMFunc
  Bus Selector1 : BusSelector  OutputSignals=rv,OperationState
  Bus Selector2 : BusSelector  OutputSignals=Func_used.OSMFunc_PowerOn
  Constant : Constant  Value=2
  Constant1 : Constant  Value=3
  Demux : Demux  Outputs=2
  Mux : Mux  Inputs=2
  Mux1 : Mux  Inputs=2
  OSMFunc_PowerOn : Constant  Value=4
  Signal Conversion : SignalConversion  ConversionOutput=Bus copy  OverrideOpt=off
  Switch : Switch  Criteria=u2 ~= 0
  Bus Out : Outport
  wires:
  Bus In/1 -> Bus Selector/1, Bus Selector1/1
  Bus Creator/1 -> Signal Conversion/1
  Input/1 -> Bus Selector2/1
  Switch/1 -> Demux/1
  Mux/1 -> Switch/3
  Bus Selector/1 -> Mux/1  "<OSMFunc>"
  Constant1/1 -> Mux/2
  Bus Selector1/1 -> Bus Creator/1  "<rv>"
  Signal Conversion/1 -> Bus Out/1
  Bus Selector1/2 -> Bus Creator/2  "<OperationState>"
  Demux/1 -> Bus Creator/3  "OSMFunc"
  Demux/2 -> Bus Creator/4  "State"
  Bus Selector2/1 -> Switch/2  "<OSMFunc_PowerOn>"
  Mux1/1 -> Switch/1
  OSMFunc_PowerOn/1 -> Mux1/1
  Constant/1 -> Mux1/2

== system MyPTControlOSM_RTW/MyPTControlOSM/PowerAcc/PowerOn reached ==
  Bus In : Inport
  State 3 PowerOn reached : ActionPort  ActionType=default
  Bus Creator : BusCreator  Inputs=4
  Bus Selector2 : BusSelector  OutputSignals=OSMFunc,State
  Constant : Constant
  OperState_PowerOn : Constant  Value=3
  Signal Conversion : SignalConversion  ConversionOutput=Bus copy  OverrideOpt=off
  Bus Out : Outport
  wires:
  Signal Conversion/1 -> Bus Out/1
  Bus Selector2/2 -> Bus Creator/4  "<State>"
  Bus Selector2/1 -> Bus Creator/3  "<OSMFunc>"
  OperState_PowerOn/1 -> Bus Creator/2  "OperationState"
  Constant/1 -> Bus Creator/1  "rv"
  Bus Creator/1 -> Signal Conversion/1
  Bus In/1 -> Bus Selector2/1

== system MyPTControlOSM_RTW/MyPTControlOSM/PowerAcc/Wait for PowerOn is ready ==
  Bus In : Inport
  Input : Inport  Port=2
  State 2 Wait for PowerOn is ready : ActionPort  ActionType=case
  Bus Assignment : BusAssignment  AssignedSignals=State
  Bus Selector : BusSelector  OutputSignals=FuncReturn
  Constant : Constant  Value=3
  Constant1 : Constant  Value=2
  Signal Conversion : SignalConversion  ConversionOutput=Bus copy  OverrideOpt=off
  Switch : Switch  Criteria=u2 ~= 0
  Bus Out : Outport
  wires:
  Signal Conversion/1 -> Bus Out/1
  Bus Assignment/1 -> Signal Conversion/1
  Bus In/1 -> Bus Assignment/1
  Input/1 -> Bus Selector/1
  Bus Selector/1 -> Switch/2  "<FuncReturn>"
  Constant/1 -> Switch/1
  Constant1/1 -> Switch/3
  Switch/1 -> Bus Assignment/2

== system MyPTControlOSM_RTW/MyPTControlOSM/PowerOff/PowerAcc function exist? ==
  Bus In : Inport
  Input : Inport  Port=2
  State 1 PowerAcc function exist? : ActionPort  ActionType=case
  Bus Creator : BusCreator  Inputs=4
  Bus Selector : BusSelector  OutputSignals=OSMFunc
  Bus Selector1 : BusSelector  OutputSignals=rv,OperationState
  Bus Selector2 : BusSelector  OutputSignals=Func_used.OSMFunc_PowerAcc
  Constant : Constant  Value=2
  Constant1 : Constant  Value=3
  Demux : Demux  Outputs=2
  Mux : Mux  Inputs=2
  Mux1 : Mux  Inputs=2
  OSMFunc_PowerAcc : Constant  Value=2
  Signal Conversion : SignalConversion  ConversionOutput=Bus copy  OverrideOpt=off
  Switch : Switch  Criteria=u2 ~= 0
  Bus Out : Outport
  wires:
  Bus In/1 -> Bus Selector/1, Bus Selector1/1
  Bus Creator/1 -> Signal Conversion/1
  Input/1 -> Bus Selector2/1
  Switch/1 -> Demux/1
  Mux/1 -> Switch/3
  Bus Selector/1 -> Mux/1  "<OSMFunc>"
  Constant1/1 -> Mux/2
  Bus Selector1/1 -> Bus Creator/1  "<rv>"
  Signal Conversion/1 -> Bus Out/1
  Bus Selector1/2 -> Bus Creator/2  "<OperationState>"
  Demux/1 -> Bus Creator/3  "OSMFunc"
  Demux/2 -> Bus Creator/4  "State"
  Bus Selector2/1 -> Switch/2  "<OSMFunc_PowerAcc>"
  Mux1/1 -> Switch/1
  OSMFunc_PowerAcc/1 -> Mux1/1
  Constant/1 -> Mux1/2

== system MyPTControlOSM_RTW/MyPTControlOSM/PowerOff/PowerAcc ready ==
  Bus In : Inport
  State 3 PowerAcc reached : ActionPort  ActionType=default
  Bus Creator : BusCreator  Inputs=4
  Bus Selector2 : BusSelector  OutputSignals=OSMFunc,State
  Constant : Constant
  OperState_PowerAccessory : Constant  Value=2
  Signal Conversion : SignalConversion  ConversionOutput=Bus copy  OverrideOpt=off
  Bus Out : Outport
  wires:
  Signal Conversion/1 -> Bus Out/1
  Bus Selector2/2 -> Bus Creator/4  "<State>"
  Bus Selector2/1 -> Bus Creator/3  "<OSMFunc>"
  OperState_PowerAccessory/1 -> Bus Creator/2  "OperationState"
  Constant/1 -> Bus Creator/1  "rv"
  Bus Creator/1 -> Signal Conversion/1
  Bus In/1 -> Bus Selector2/1

== system MyPTControlOSM_RTW/MyPTControlOSM/PowerOff/PowerOff -> PowerAcc? ==
  Bus In : Inport
  Input : Inport  Port=2
  "State 0 PowerOff -> PowerAcc?" : ActionPort  ActionType=case
  >= KeyIn_PowerAcc : simulink/Logic and Bit Operations/Compare To Constant  SystemSampleTime=-1  relop=>=  const=2  LogicOutDataTypeMode=uint8  ZeroCross=off
  Bus Assignment : BusAssignment  AssignedSignals=State
  Bus Selector : BusSelector  OutputSignals=Key
  Constant : Constant
  Constant1 : Constant  Value=0
  Signal Conversion : SignalConversion  ConversionOutput=Bus copy  OverrideOpt=off
  Switch : Switch  Criteria=u2 ~= 0
  Bus Out : Outport
  wires:
  Bus In/1 -> Bus Assignment/1
  Bus Assignment/1 -> Signal Conversion/1
  Signal Conversion/1 -> Bus Out/1
  Switch/1 -> Bus Assignment/2
  Input/1 -> Bus Selector/1
  Bus Selector/1 -> >= KeyIn_PowerAcc/1  "<Key>"
  Constant/1 -> Switch/1
  Constant1/1 -> Switch/3
  >= KeyIn_PowerAcc/1 -> Switch/2

== system MyPTControlOSM_RTW/MyPTControlOSM/PowerOff/Wait for PowerAcc is ready ==
  Bus In : Inport
  Input : Inport  Port=2
  State 2 Wait for PowerAcc is ready : ActionPort  ActionType=case
  Bus Assignment : BusAssignment  AssignedSignals=State
  Bus Selector : BusSelector  OutputSignals=FuncReturn
  Constant : Constant  Value=3
  Constant1 : Constant  Value=2
  Signal Conversion : SignalConversion  ConversionOutput=Bus copy  OverrideOpt=off
  Switch : Switch  Criteria=u2 ~= 0
  Bus Out : Outport
  wires:
  Signal Conversion/1 -> Bus Out/1
  Bus Assignment/1 -> Signal Conversion/1
  Bus In/1 -> Bus Assignment/1
  Input/1 -> Bus Selector/1
  Bus Selector/1 -> Switch/2  "<FuncReturn>"
  Constant/1 -> Switch/1
  Constant1/1 -> Switch/3
  Switch/1 -> Bus Assignment/2

== system MyPTControlOSM_RTW/MyPTControlOSM/PowerOn/Drive reached ==
  Bus In : Inport
  State 3 Drive reached : ActionPort  ActionType=case
  Bus Creator1 : BusCreator  Inputs=4
  Bus Selector4 : BusSelector  OutputSignals=OSMFunc,State
  Constant : Constant
  OperState_Driving : Constant  Value=4
  Signal Conversion : SignalConversion  ConversionOutput=Bus copy  OverrideOpt=off
  Bus Out : Outport
  wires:
  Signal Conversion/1 -> Bus Out/1
  Bus Selector4/2 -> Bus Creator1/4  "<State>"
  Bus Selector4/1 -> Bus Creator1/3  "<OSMFunc>"
  OperState_Driving/1 -> Bus Creator1/2  "OperationState"
  Constant/1 -> Bus Creator1/1  "rv"
  Bus Creator1/1 -> Signal Conversion/1
  Bus In/1 -> Bus Selector4/1

== system MyPTControlOSM_RTW/MyPTControlOSM/PowerOn/PowerOff function exist? ==
  Bus In : Inport
  Input : Inport  Port=2
  State 9 PowerOff function exist? : ActionPort  ActionType=case
  Bus Creator : BusCreator  Inputs=4
  Bus Selector1 : BusSelector  OutputSignals=OSMFunc
  Bus Selector2 : BusSelector  OutputSignals=rv,OperationState
  Bus Selector3 : BusSelector  OutputSignals=Func_used.OSMFunc_PowerOff
  Constant2 : Constant  Value=8
  Constant3 : Constant  Value=11
  Demux : Demux  Outputs=2
  Mux : Mux  Inputs=2
  Mux1 : Mux  Inputs=2
  OSMFunc_PowerOff : Constant  Value=2
  Signal Conversion : SignalConversion  ConversionOutput=Bus copy  OverrideOpt=off
  Switch1 : Switch  Criteria=u2 ~= 0
  Bus Out : Outport
  wires:
  Bus In/1 -> Bus Selector1/1, Bus Selector2/1
  Bus Creator/1 -> Signal Conversion/1
  Input/1 -> Bus Selector3/1
  Switch1/1 -> Demux/1
  Mux/1 -> Switch1/3
  Bus Selector1/1 -> Mux/1  "<OSMFunc>"
  Constant3/1 -> Mux/2  "State"
  Signal Conversion/1 -> Bus Out/1
  Bus Selector2/2 -> Bus Creator/2  "<OperationState>"
  Demux/1 -> Bus Creator/3  "OSMFunc"
  Demux/2 -> Bus Creator/4  "State"
  Bus Selector3/1 -> Switch1/2  "<OSMFunc_PowerOff>"
  Bus Selector2/1 -> Bus Creator/1  "<rv>"
  Constant2/1 -> Mux1/2  "State"
  OSMFunc_PowerOff/1 -> Mux1/1
  Mux1/1 -> Switch1/1

== system MyPTControlOSM_RTW/MyPTControlOSM/PowerOn/PowerOff reached ==
  Bus In : Inport
  State 11 PowerOff reached : ActionPort  ActionType=default
  Bus Creator1 : BusCreator  Inputs=4
  Bus Selector4 : BusSelector  OutputSignals=OSMFunc,State
  Constant : Constant
  OperState_PowerOff : Constant
  Signal Conversion : SignalConversion  ConversionOutput=Bus copy  OverrideOpt=off
  Bus Out : Outport
  wires:
  Signal Conversion/1 -> Bus Out/1
  Bus Selector4/2 -> Bus Creator1/4  "<State>"
  Bus Selector4/1 -> Bus Creator1/3  "<OSMFunc>"
  OperState_PowerOff/1 -> Bus Creator1/2  "OperationState"
  Constant/1 -> Bus Creator1/1  "rv"
  Bus Creator1/1 -> Signal Conversion/1
  Bus In/1 -> Bus Selector4/1

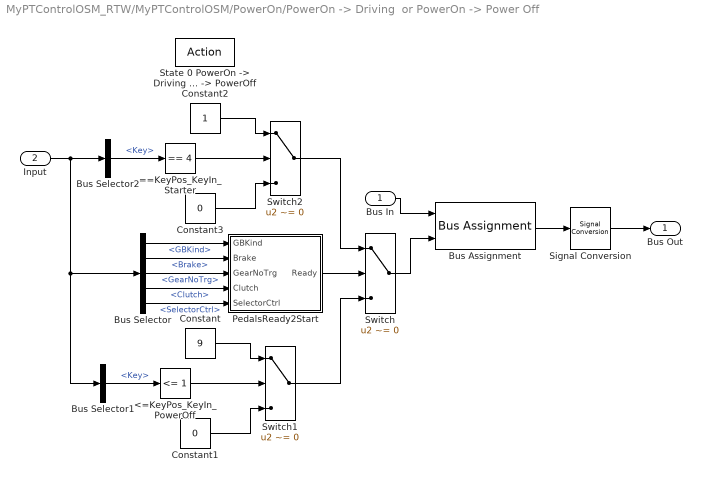
== system MyPTControlOSM_RTW/MyPTControlOSM/PowerOn/PowerOn -> Driving  or PowerOn -> Power Off ==
  Bus In : Inport
  Input : Inport  Port=2
  "State 0 PowerOn -> Driving or PowerOn -> PowerOff" : ActionPort  ActionType=case
  <=KeyPos_KeyIn_PowerOff : simulink/Logic and Bit Operations/Compare To Constant  SystemSampleTime=-1  relop=<=  const=1  LogicOutDataTypeMode=uint8  ZeroCross=off
  ==KeyPos_KeyIn_Starter : simulink/Logic and Bit Operations/Compare To Constant  SystemSampleTime=-1  relop===  const=4  LogicOutDataTypeMode=uint8  ZeroCross=off
  Bus Assignment : BusAssignment  AssignedSignals=State
  Bus Selector : BusSelector  OutputSignals=GBKind,Brake,GearNoTrg,Clutch,SelectorCtrl
  Bus Selector1 : BusSelector  OutputSignals=Key
  Bus Selector2 : BusSelector  OutputSignals=Key
  Constant : Constant  Value=9
  Constant1 : Constant  Value=0
  Constant2 : Constant
  Constant3 : Constant  Value=0
  PedalsReady2Start : Subsystem
  Signal Conversion : SignalConversion  ConversionOutput=Bus copy  OverrideOpt=off
  Switch : Switch  Criteria=u2 ~= 0
  Switch1 : Switch  Criteria=u2 ~= 0
  Switch2 : Switch  Criteria=u2 ~= 0
  Bus Out : Outport
  wires:
  Bus Assignment/1 -> Signal Conversion/1
  Signal Conversion/1 -> Bus Out/1
  Bus In/1 -> Bus Assignment/1
  Switch1/1 -> Switch/3
  Switch/1 -> Bus Assignment/2
  <=KeyPos_KeyIn_PowerOff/1 -> Switch1/2
  Constant/1 -> Switch1/1
  Constant1/1 -> Switch1/3
  Input/1 -> Bus Selector1/1, Bus Selector/1, Bus Selector2/1
  Bus Selector1/1 -> <=KeyPos_KeyIn_PowerOff/1  "<Key>"
  ==KeyPos_KeyIn_Starter/1 -> Switch2/2
  Constant2/1 -> Switch2/1
  Constant3/1 -> Switch2/3
  Bus Selector2/1 -> ==KeyPos_KeyIn_Starter/1  "<Key>"
  Switch2/1 -> Switch/1
  PedalsReady2Start/1(Ready) -> Switch/2
  Bus Selector/1 -> PedalsReady2Start/1(GBKind)  "<GBKind>"
  Bus Selector/2 -> PedalsReady2Start/2(Brake)  "<Brake>"
  Bus Selector/3 -> PedalsReady2Start/3(GearNoTrg)  "<GearNoTrg>"
  Bus Selector/4 -> PedalsReady2Start/4(Clutch)  "<Clutch>"
  Bus Selector/5 -> PedalsReady2Start/5(SelectorCtrl)  "<SelectorCtrl>"

== system MyPTControlOSM_RTW/MyPTControlOSM/PowerOn/PowerOn reached -> back to beginning ==
  Bus In : Inport
  "State 8 PowerOn reached -> back to beginning" : ActionPort  ActionType=case
  Bus Creator1 : BusCreator  Inputs=4
  Bus Selector4 : BusSelector  OutputSignals=OSMFunc,State
  Constant : Constant
  OperState_PowerOn : Constant  Value=3
  Signal Conversion : SignalConversion  ConversionOutput=Bus copy  OverrideOpt=off
  Bus Out : Outport
  wires:
  Signal Conversion/1 -> Bus Out/1
  Bus Selector4/2 -> Bus Creator1/4  "<State>"
  Bus Selector4/1 -> Bus Creator1/3  "<OSMFunc>"
  OperState_PowerOn/1 -> Bus Creator1/2  "OperationState"
  Constant/1 -> Bus Creator1/1  "rv"
  Bus Creator1/1 -> Signal Conversion/1
  Bus In/1 -> Bus Selector4/1

== system MyPTControlOSM_RTW/MyPTControlOSM/PowerOn/SkipStart function exist? ==
  Bus In : Inport
  Input : Inport  Port=2
  State 4 SkipStart function exist? : ActionPort  ActionType=case
  Bus Creator : BusCreator  Inputs=4
  Bus Selector1 : BusSelector  OutputSignals=OSMFunc
  Bus Selector2 : BusSelector  OutputSignals=rv,OperationState
  Bus Selector3 : BusSelector  OutputSignals=Func_used.OSMFunc_SkipStart
  Constant2 : Constant  Value=5
  Constant3 : Constant  Value=6
  Demux : Demux  Outputs=2
  Mux : Mux  Inputs=2
  Mux1 : Mux  Inputs=2
  OSMFunc_SkipStart : Constant  Value=6
  Signal Conversion : SignalConversion  ConversionOutput=Bus copy  OverrideOpt=off
  Switch1 : Switch  Criteria=u2 ~= 0
  Bus Out : Outport
  wires:
  Bus In/1 -> Bus Selector1/1, Bus Selector2/1
  Bus Creator/1 -> Signal Conversion/1
  Input/1 -> Bus Selector3/1
  Switch1/1 -> Demux/1
  Mux/1 -> Switch1/3
  Bus Selector1/1 -> Mux/1  "<OSMFunc>"
  Constant3/1 -> Mux/2  "State"
  Signal Conversion/1 -> Bus Out/1
  Bus Selector2/2 -> Bus Creator/2  "<OperationState>"
  Demux/1 -> Bus Creator/3  "OSMFunc"
  Demux/2 -> Bus Creator/4  "State"
  Bus Selector3/1 -> Switch1/2  "<OSMFunc_SkipStart>"
  Bus Selector2/1 -> Bus Creator/1  "<rv>"
  Constant2/1 -> Mux1/2  "State"
  OSMFunc_SkipStart/1 -> Mux1/1
  Mux1/1 -> Switch1/1

== system MyPTControlOSM_RTW/MyPTControlOSM/PowerOn/SkipStart reached -> PowerOn function exist? ==
  Bus In : Inport
  Input : Inport  Port=2
  "State 6 SkipStart reached -> PowerOn function exist?" : ActionPort  ActionType=case
  Bus Creator : BusCreator  Inputs=4
  Bus Selector1 : BusSelector  OutputSignals=OSMFunc
  Bus Selector2 : BusSelector  OutputSignals=rv,OperationState
  Bus Selector3 : BusSelector  OutputSignals=Func_used.OSMFunc_PowerOn
  Constant2 : Constant  Value=7
  Constant3 : Constant  Value=8
  Demux : Demux  Outputs=2
  Mux : Mux  Inputs=2
  Mux1 : Mux  Inputs=2
  OSMFunc_PowerOn : Constant  Value=4
  Signal Conversion1 : SignalConversion  ConversionOutput=Bus copy  OverrideOpt=off
  Switch1 : Switch  Criteria=u2 ~= 0
  Bus Out : Outport
  wires:
  Bus In/1 -> Bus Selector1/1, Bus Selector2/1
  Bus Creator/1 -> Signal Conversion1/1
  Input/1 -> Bus Selector3/1
  Switch1/1 -> Demux/1
  Mux/1 -> Switch1/3
  Bus Selector1/1 -> Mux/1  "<OSMFunc>"
  Constant3/1 -> Mux/2  "State"
  Signal Conversion1/1 -> Bus Out/1
  Bus Selector2/2 -> Bus Creator/2  "<OperationState>"
  Demux/1 -> Bus Creator/3  "OSMFunc"
  Demux/2 -> Bus Creator/4  "State"
  Bus Selector3/1 -> Switch1/2  "<OSMFunc_PowerOn>"
  Bus Selector2/1 -> Bus Creator/1  "<rv>"
  Constant2/1 -> Mux1/2  "State"
  OSMFunc_PowerOn/1 -> Mux1/1
  Mux1/1 -> Switch1/1

== system MyPTControlOSM_RTW/MyPTControlOSM/PowerOn/Start function exist? ==
  Bus In : Inport
  Input : Inport  Port=2
  State 1 Start function exist? : ActionPort  ActionType=case
  Bus Creator : BusCreator  Inputs=4
  Bus Selector1 : BusSelector  OutputSignals=OSMFunc
  Bus Selector2 : BusSelector  OutputSignals=rv,OperationState
  Bus Selector3 : BusSelector  OutputSignals=Func_used.OSMFunc_SkipStart
  Constant2 : Constant  Value=2
  Constant3 : Constant  Value=3
  Demux : Demux  Outputs=2
  Mux : Mux  Inputs=2
  Mux1 : Mux  Inputs=2
  OSMFunc_Start : Constant  Value=5
  Signal Conversion1 : SignalConversion  ConversionOutput=Bus copy  OverrideOpt=off
  Switch1 : Switch  Criteria=u2 ~= 0
  Bus Out : Outport
  wires:
  Bus In/1 -> Bus Selector1/1, Bus Selector2/1
  Bus Creator/1 -> Signal Conversion1/1
  Input/1 -> Bus Selector3/1
  Switch1/1 -> Demux/1
  Mux/1 -> Switch1/3
  Bus Selector1/1 -> Mux/1  "<OSMFunc>"
  Constant3/1 -> Mux/2  "State"
  Signal Conversion1/1 -> Bus Out/1
  Bus Selector2/2 -> Bus Creator/2  "<OperationState>"
  Demux/1 -> Bus Creator/3  "OSMFunc"
  Demux/2 -> Bus Creator/4  "State"
  Bus Selector3/1 -> Switch1/2  "<OSMFunc_SkipStart>"
  Constant2/1 -> Mux1/2  "State"
  OSMFunc_Start/1 -> Mux1/1
  Mux1/1 -> Switch1/1
  Bus Selector2/1 -> Bus Creator/1  "<rv>"

== system MyPTControlOSM_RTW/MyPTControlOSM/PowerOn/Wait for PowerOff is ready ==
  Bus In : Inport
  Input : Inport  Port=2
  State 10 Wait for PowerOff is ready : ActionPort  ActionType=case
  Bus Assignment : BusAssignment  AssignedSignals=State
  Bus Selector : BusSelector  OutputSignals=FuncReturn
  Constant : Constant  Value=11
  Constant1 : Constant  Value=10
  Signal Conversion : SignalConversion  ConversionOutput=Bus copy  OverrideOpt=off
  Switch : Switch  Criteria=u2 ~= 0
  Bus Out : Outport
  wires:
  Signal Conversion/1 -> Bus Out/1
  Bus Assignment/1 -> Signal Conversion/1
  Bus In/1 -> Bus Assignment/1
  Input/1 -> Bus Selector/1
  Bus Selector/1 -> Switch/2  "<FuncReturn>"
  Constant/1 -> Switch/1
  Constant1/1 -> Switch/3
  Switch/1 -> Bus Assignment/2

== system MyPTControlOSM_RTW/MyPTControlOSM/PowerOn/Wait for PowerOn is ready ==
  Bus In : Inport
  Input : Inport  Port=2
  State 7 Wait for PowerOn is ready : ActionPort  ActionType=case
  Bus Assignment : BusAssignment  AssignedSignals=State
  Bus Selector : BusSelector  OutputSignals=FuncReturn
  Constant : Constant  Value=8
  Constant1 : Constant  Value=7
  Signal Conversion : SignalConversion  ConversionOutput=Bus copy  OverrideOpt=off
  Switch : Switch  Criteria=u2 ~= 0
  Bus Out : Outport
  wires:
  Signal Conversion/1 -> Bus Out/1
  Bus Assignment/1 -> Signal Conversion/1
  Bus In/1 -> Bus Assignment/1
  Input/1 -> Bus Selector/1
  Bus Selector/1 -> Switch/2  "<FuncReturn>"
  Constant/1 -> Switch/1
  Constant1/1 -> Switch/3
  Switch/1 -> Bus Assignment/2

== system MyPTControlOSM_RTW/MyPTControlOSM/PowerOn/Wait for SkipStart is ready ==
  Bus In : Inport
  Input : Inport  Port=2
  State 5 Wait for SkipStart is ready : ActionPort  ActionType=case
  Bus Assignment : BusAssignment  AssignedSignals=State
  Bus Selector : BusSelector  OutputSignals=FuncReturn
  Constant : Constant  Value=6
  Constant1 : Constant  Value=5
  Signal Conversion : SignalConversion  ConversionOutput=Bus copy  OverrideOpt=off
  Switch : Switch  Criteria=u2 ~= 0
  Bus Out : Outport
  wires:
  Signal Conversion/1 -> Bus Out/1
  Bus Assignment/1 -> Signal Conversion/1
  Bus In/1 -> Bus Assignment/1
  Input/1 -> Bus Selector/1
  Bus Selector/1 -> Switch/2  "<FuncReturn>"
  Constant/1 -> Switch/1
  Constant1/1 -> Switch/3
  Switch/1 -> Bus Assignment/2
